simulink model "helicopter_NN_ports"  (R2019a)
settings: Solver=FixedStepAuto  StartTime=0.0  StopTime=4.0  FixedStep=0.01  RelTol=1e-3
values from neighbouring files (symbols this model uses):
  a = 1    [run_nk_helicopter.m]
  i = 0    [run_nk_helicopter.m]
  K = 10    [run_nk_helicopter.m]
undefined symbols (not defined in the file or in its folder): options
libraries: neural x66, simulink x2
(part 3 of 3)

== system helicopter_NN_ports/Feed-Forward Neural Network/Layer 3/Delays 1 ==
  "p{3}" : Inport  PortDimensions=30
      mask Display: e = 0.06;c1 = [120 230 180]/255;c2 = ([120 230 180]+0)/(256+128);c3 = ([120 230 180]+128)/(256+128);patch([0 1 1 0],[0 0 1 1],c1);patch([0 1 1 1-e 1-e 0+e],[0 0 1 1-e 0+e 0+e],c2);patch([0 0 1 1-e 0+e 0+e],[0 1 1 1-e 1-e 0+e],c3);plot([0 1 1 0 0],[0 0 1 1 0]);
  mux : Mux  Inputs=1
      mask Display: e = 0.06;c1 = [120 150 230]/255;c2 = ([120 150 230]+0)/383;c3 = ([120 150 230]+128)/383;patch([0 1 1 0],[0 0 1 1],c1);patch([0 1 1 1-e 1-e 0+e],[0 0 1 1-e 0+e 0+e],c2);patch([0 0 1 1-e 0+e 0+e],[0 1 1 1-e 1-e 0+e],c3);plot([0 1 1 0 0],[0 0 1 1 0]);disp('Mux')
  "pd{3,2}" : Outport
      mask Display: e = 0.06;c1 = [120 230 180]/255;c2 = ([120 230 180]+0)/(256+128);c3 = ([120 230 180]+128)/(256+128);patch([0 1 1 0],[0 0 1 1],c1);patch([0 1 1 1-e 1-e 0+e],[0 0 1 1-e 0+e 0+e],c2);patch([0 0 1 1-e 0+e 0+e],[0 1 1 1-e 1-e 0+e],c3);plot([0 1 1 0 0],[0 0 1 1 0]);
  wires:
  "p{3}"/1 -> mux/1
  mux/1 -> "pd{3,2}"/1

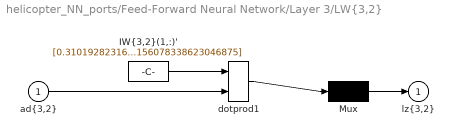
== system helicopter_NN_ports/Feed-Forward Neural Network/Layer 3/LW{3,2} ==
  "ad{3,2}" : Inport  PortDimensions=30
      mask Display: e = 0.06;c1 = [120 230 180]/255;c2 = ([120 230 180]+0)/(256+128);c3 = ([120 230 180]+128)/(256+128);patch([0 1 1 0],[0 0 1 1],c1);patch([0 1 1 1-e 1-e 0+e],[0 0 1 1-e 0+e 0+e],c2);patch([0 0 1 1-e 0+e 0+e],[0 1 1 1-e 1-e 0+e],c3);plot([0 1 1 0 0],[0 0 1 1 0]);
  "IW{3,2}(1,:)'" : Constant  Value=[0.31019282316940877120003960953908972442150115966796875;0.1105061913110494675738237901896354742348194122314453125;-0.240315269054316382746350200250162743031978607177734375;-0.34132182292024226821780530372052453458309173583984375;-0.324785581712588200531399706960655748844146728515625;0.190601643960655431353501398916705511510372161865234375;0.06776909021280363987216333043761551380157470703125;-0.08333443917583273352622796892319456674158573150634765625;0.2027827723003554349912036514069768600165843963623046875;0.289413618170612618740733523736707866191864013671875;-0.07200489663712590637789645597877097316086292266845703125;0.162858859106621400858472270556376315653324127197265625;-0.1790762756517174925097179993827012367546558380126953125;0.304763020541672313701297980514937080442905426025390625;-0.515272988938287657134651453816331923007965087890625;0.283941674837810797971116016924497671425342559814453125;0.1147428522126223982002812817881931550800800323486328125;0.385476380895737935627920478509622626006603240966796875;0.0752312546095022238734628672318649478256702423095703125;-0.25668576925872310656728814137750305235385894775390625;0.2220252388767010309766902764749829657375812530517578125;-0.32064049099083946625654562012641690671443939208984375;0.1673564997460565695330814151020604185760021209716796875;0.2859765994810266054315661676810123026371002197265625;-0.381351669210497068451815039225039072334766387939453125;0.2059759080325982705250709159372490830719470977783203125;-0.2116925143613337112480365931332926265895366668701171875;-0.392627904588735254787223993844236247241497039794921875;-0.294750981722224747461069682685774751007556915283203125;0.131153047345179796234759805884095840156078338623046875]
      mask Display: e = 0.06;c1 = [120 150 230]/255;c2 = ([120 150 230]+0)/383;c3 = ([120 150 230]+128)/383;patch([0 1 1 0],[0 0 1 1],c1);patch([0 1 1 1-e 1-e 0+e],[0 0 1 1-e 0+e 0+e],c2);patch([0 0 1 1-e 0+e 0+e],[0 1 1 1-e 1-e 0+e],c3);plot([0 1 1 0 0],[0 0 1 1 0]);disp('weights');
  Mux : Mux  Inputs=1
      mask Display: e = 0.06;c1 = [120 150 230]/255;c2 = ([120 150 230]+0)/383;c3 = ([120 150 230]+128)/383;patch([0 1 1 0],[0 0 1 1],c1);patch([0 1 1 1-e 1-e 0+e],[0 0 1 1-e 0+e 0+e],c2);patch([0 0 1 1-e 0+e 0+e],[0 1 1 1-e 1-e 0+e],c3);plot([0 1 1 0 0],[0 0 1 1 0]);disp('Mux');
  dotprod1 : neural/Weight Functions/dotprod
      settings: SourceProductName=Deep Learning Toolbox
  "lz{3,2}" : Outport
      mask Display: e = 0.06;c1 = [120 230 180]/255;c2 = ([120 230 180]+0)/(256+128);c3 = ([120 230 180]+128)/(256+128);patch([0 1 1 0],[0 0 1 1],c1);patch([0 1 1 1-e 1-e 0+e],[0 0 1 1-e 0+e 0+e],c2);patch([0 0 1 1-e 0+e 0+e],[0 1 1 1-e 1-e 0+e],c3);plot([0 1 1 0 0],[0 0 1 1 0]);
  wires:
  "IW{3,2}(1,:)'"/1 -> dotprod1/1
  "ad{3,2}"/1 -> dotprod1/2
  dotprod1/1 -> Mux/1
  Mux/1 -> "lz{3,2}"/1
